simulink model "remote"  (Simulink 7.6)
settings: Solver=ode5  StartTime=0.0  StopTime=10.0  FixedStep=Ts  RelTol=1e-3
values from neighbouring files (symbols this model uses):
  g = 9.8065    [kostas_malakies.mat]    (also in kostas_malakies2.mat; load_PMModel.m = 9.81; main.m; main_last.m)
  mass = 0.66    [kostas_malakies.mat]    (also in kostas_malakies2.mat; load_PMModel.m = 0.687; main_last.m)
  N = 5    [matlab.mat]
  Ts = 0.02    [kostas_malakies.mat]    (also in kostas_malakies2.mat; main.m; main_last.m; matlab.mat = 0.08)
  Ts_slow = 0.02    [kostas_malakies.mat]    (also in kostas_malakies2.mat; main.m; main_last.m)
  yaw0 = 0    [kostas_malakies.mat]    (also in kostas_malakies2.mat; main.m; main_last.m; matlab.mat = -0.0873)
undefined symbols (not defined in the file or in its folder): AA_delay_x, AA_delay_y, AA_delay_yaw, AA_delay_z, BB_delay_x, BB_delay_y, BB_delay_yaw, BB_delay_z, betas_x, betas_y, betas_yaw, betas_z, delay_steps_x, delay_steps_y, delay_steps_yaw, delay_steps_z, i_min_cs_pre_rough_x, i_min_cs_pre_rough_y, i_min_cs_pre_rough_yaw, i_min_cs_pre_rough_z, kalmf_bias_x, kalmf_bias_y, kalmf_bias_z, L_x, L_y, L_yaw, L_z, LL_PP_x, LL_PP_y, LL_PP_yaw, LL_PP_z, LL_ref_PP_x, LL_ref_PP_y, LL_ref_PP_yaw, LL_ref_PP_z, MM_x, MM_y, MM_yaw, MM_z, PP_x, PP_y, PP_yaw, PP_z, TT_PP_x, TT_PP_y, TT_PP_yaw, TT_PP_z, V_max_x, V_max_y, V_max_yaw, V_max_z
libraries: simulink x18, Hqaud_model_LIB_SI x5, Hquad_control_LIB_SI x1
(part 1 of 2)
settings Model: Creator=burrimi  LastModifiedBy=burrimi
settings DataIOCC: SaveOutput=off  SaveTime=off
settings OptimizationCC: ZeroExternalMemoryAtStartup=off  OptimizeModelRefInitCode=on  LifeSpan=1
settings HardwareCC: ProdIntDivRoundTo=Zero  ProdEndianess=LittleEndian  ProdHWDeviceType=Intel Pentium  TargetIntDivRoundTo=Zero  TargetEndianess=LittleEndian  TargetHWDeviceType=MATLAB Host
settings RTWCC: SystemTargetFile=ert.tlc  TemplateMakefile=ert_default_tmf  Description=Real-Time Workshop Embedded Coder  GenerateReport=on  ProcessScript=ert_make_rtw_hook  IncludeHyperlinkInReport=on  LaunchReport=on  TargetLang=C++ (Encapsulated)
settings ERTTargetCC: MultiwordLength=2048  GenerateSampleERTMain=on  MultiInstanceERTCode=on  SupportContinuousTime=on  RootIOFormat=Structure reference  ERTCustomFileTemplate=example_file_process.tlc  ConvertIfToSwitch=off
settings ERTCPPComponent: GenerateDestructor=on  GenerateExternalIOAccessMethods=None  ParameterMemberVisibility=private  InternalMemberVisibility=private  GenerateParameterAccessMethods=None  GenerateInternalMemberAccessMethods=None  UseOperatorNewForModelRefRegistration=off

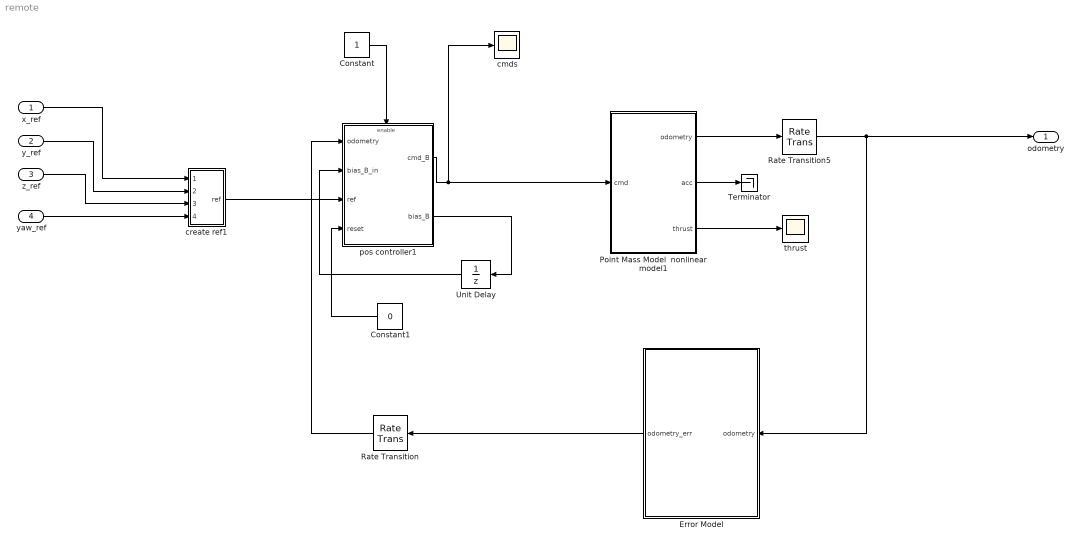
== system remote ==
  x_ref : Inport  PortDimensions=1  SampleTime=Ts
  y_ref : Inport  Port=2  PortDimensions=1  SampleTime=Ts
  z_ref : Inport  Port=3  PortDimensions=1  SampleTime=Ts
  yaw_ref : Inport  Port=4  PortDimensions=1  SampleTime=Ts
  Constant : Constant
  Constant1 : Constant  Value=0
  Error Model : Subsystem
  Point Mass Model  nonlinear model1 : Subsystem  AncestorBlock="Hqaud_model_LIB_SI/Point Mass Model  nonlinear model"
  Rate Transition : RateTransition  OutPortSampleTime=Ts
  Rate Transition5 : RateTransition  OutPortSampleTime=Ts_slow
  Terminator : Terminator
  Unit Delay : UnitDelay  SampleTime=-1
  cmds : Scope
      settings: TimeRange=39.996  YMin=-3  YMax=1
  create ref1 : Subsystem
  pos controller1 : Subsystem  AncestorBlock=Hquad_control_LIB_SI/pos controller
  thrust : Scope
      settings: TimeRange=40  YMin=113.9130434782609  YMax=138.2608695652174
  odometry : Outport  SampleTime=Ts
  wires:
  Point Mass Model  nonlinear model1/3("thrust   ") -> thrust/1
  pos controller1/1(cmd_B) -> cmds/1, Point Mass Model  nonlinear model1/1(cmd)
  Constant/1 -> pos controller1/Enable
  Point Mass Model  nonlinear model1/2(acc) -> Terminator/1
  Constant1/1 -> pos controller1/4(reset)
  Point Mass Model  nonlinear model1/1(odometry) -> Rate Transition5/1
  Rate Transition/1 -> pos controller1/1(odometry)
  Rate Transition5/1 -> odometry/1, Error Model/1(odometry)
  x_ref/1 -> create ref1/1(x_ref)
  y_ref/1 -> create ref1/2(y_ref)
  z_ref/1 -> create ref1/3(z_ref)
  yaw_ref/1 -> create ref1/4(yaw_ref)
  create ref1/1(ref) -> pos controller1/3(ref)
  pos controller1/2(bias_B) -> Unit Delay/1
  Unit Delay/1 -> pos controller1/2(bias_B_in)
  Error Model/1(odometry_err) -> Rate Transition/1

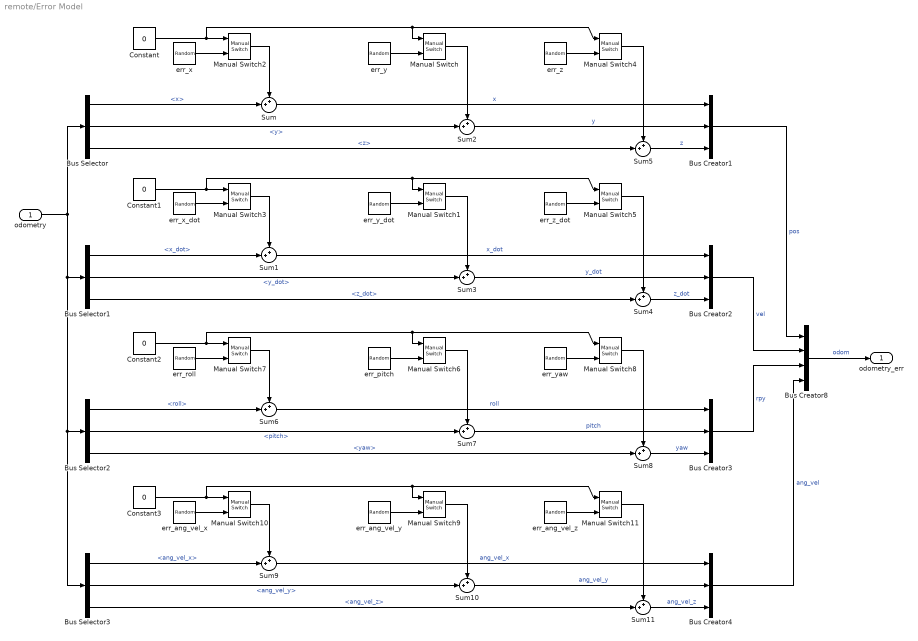
== system remote/Error Model ==
  odometry : Inport
  Bus Creator{1..4} (4 alike) : BusCreator  Inputs=3
  Bus Creator8 : BusCreator
  Bus Selector : BusSelector  OutputSignals=pos.x,pos.y,pos.z
  Bus Selector1 : BusSelector  OutputSignals=vel.x_dot,vel.y_dot,vel.z_dot
  Bus Selector2 : BusSelector  OutputSignals=rpy.roll,rpy.pitch,rpy.yaw
  Bus Selector3 : BusSelector  OutputSignals=ang_vel.ang_vel_x,ang_vel.ang_vel_y,ang_vel.ang_vel_z
  Constant{,1..3} (4 alike) : Constant  Value=0
  Manual Switch{,1..11} (12 alike) : simulink/Signal Routing/Manual Switch  SystemSampleTime=-1  sw=1  action=0  varsize=off
  Sum{,1..11} (12 alike) : Sum  Inputs=++|  SampleTime=Ts_slow
  err_ang_vel_x : RandomNumber  Variance=0.0001  SampleTime=Ts_slow
  err_ang_vel_y : RandomNumber  Variance=0.0001  SampleTime=Ts_slow
  err_ang_vel_z : RandomNumber  Variance=0.0001  SampleTime=Ts_slow
  err_pitch : RandomNumber  Variance=0.0001  SampleTime=Ts_slow
  err_roll : RandomNumber  Variance=0.0001  SampleTime=Ts_slow
  err_x : RandomNumber  Variance=0.000707  SampleTime=Ts_slow
  err_x_dot : RandomNumber  Variance=0.0001  SampleTime=Ts_slow
  err_y : RandomNumber  Variance=0.000707  SampleTime=Ts_slow
  err_y_dot : RandomNumber  Variance=0.0001  SampleTime=Ts_slow
  err_yaw : RandomNumber  Variance=0.0001  SampleTime=Ts_slow
  err_z : RandomNumber  Variance=0.000707  SampleTime=Ts_slow
  err_z_dot : RandomNumber  Variance=0.0001  SampleTime=Ts_slow
  odometry_err : Outport
  wires:
  err_z/1 -> Manual Switch4/2
  Manual Switch4/1 -> Sum5/1
  err_y/1 -> Manual Switch/2
  Manual Switch/1 -> Sum2/1
  err_x/1 -> Manual Switch2/2
  Manual Switch2/1 -> Sum/1
  Sum/1 -> Bus Creator1/1  "x"
  Bus Creator1/1 -> Bus Creator8/1  "pos"
  Sum2/1 -> Bus Creator1/2  "y"
  Sum5/1 -> Bus Creator1/3  "z"
  odometry/1 -> Bus Selector/1, Bus Selector2/1, Bus Selector3/1, Bus Selector1/1
  Bus Selector/1 -> Sum/2  "<x>"
  Bus Selector/2 -> Sum2/2  "<y>"
  Bus Selector/3 -> Sum5/2  "<z>"
  Constant/1 -> Manual Switch2/1, Manual Switch/1, Manual Switch4/1
  err_z_dot/1 -> Manual Switch5/2
  Manual Switch5/1 -> Sum4/1
  err_y_dot/1 -> Manual Switch1/2
  Manual Switch1/1 -> Sum3/1
  err_x_dot/1 -> Manual Switch3/2
  Manual Switch3/1 -> Sum1/1
  Sum1/1 -> Bus Creator2/1  "x_dot"
  Sum3/1 -> Bus Creator2/2  "y_dot"
  Sum4/1 -> Bus Creator2/3  "z_dot"
  Bus Selector1/1 -> Sum1/2  "<x_dot>"
  Bus Selector1/2 -> Sum3/2  "<y_dot>"
  Bus Selector1/3 -> Sum4/2  "<z_dot>"
  Constant1/1 -> Manual Switch3/1, Manual Switch1/1, Manual Switch5/1
  Bus Creator2/1 -> Bus Creator8/2  "vel"
  err_yaw/1 -> Manual Switch8/2
  Manual Switch8/1 -> Sum8/1
  err_pitch/1 -> Manual Switch6/2
  Manual Switch6/1 -> Sum7/1
  err_roll/1 -> Manual Switch7/2
  Manual Switch7/1 -> Sum6/1
  Sum6/1 -> Bus Creator3/1  "roll"
  Sum7/1 -> Bus Creator3/2  "pitch"
  Sum8/1 -> Bus Creator3/3  "yaw"
  Bus Selector2/1 -> Sum6/2  "<roll>"
  Bus Selector2/2 -> Sum7/2  "<pitch>"
  Bus Selector2/3 -> Sum8/2  "<yaw>"
  Constant2/1 -> Manual Switch7/1, Manual Switch6/1, Manual Switch8/1
  Bus Creator3/1 -> Bus Creator8/3  "rpy"
  err_ang_vel_z/1 -> Manual Switch11/2
  Manual Switch11/1 -> Sum11/1
  err_ang_vel_y/1 -> Manual Switch9/2
  Manual Switch9/1 -> Sum10/1
  err_ang_vel_x/1 -> Manual Switch10/2
  Manual Switch10/1 -> Sum9/1
  Sum9/1 -> Bus Creator4/1  "ang_vel_x"
  Sum10/1 -> Bus Creator4/2  "ang_vel_y"
  Sum11/1 -> Bus Creator4/3  "ang_vel_z"
  Bus Selector3/1 -> Sum9/2  "<ang_vel_x>"
  Bus Selector3/2 -> Sum10/2  "<ang_vel_y>"
  Bus Selector3/3 -> Sum11/2  "<ang_vel_z>"
  Constant3/1 -> Manual Switch10/1, Manual Switch9/1, Manual Switch11/1
  Bus Creator4/1 -> Bus Creator8/4  "ang_vel"
  Bus Creator8/1 -> odometry_err/1  "odom"

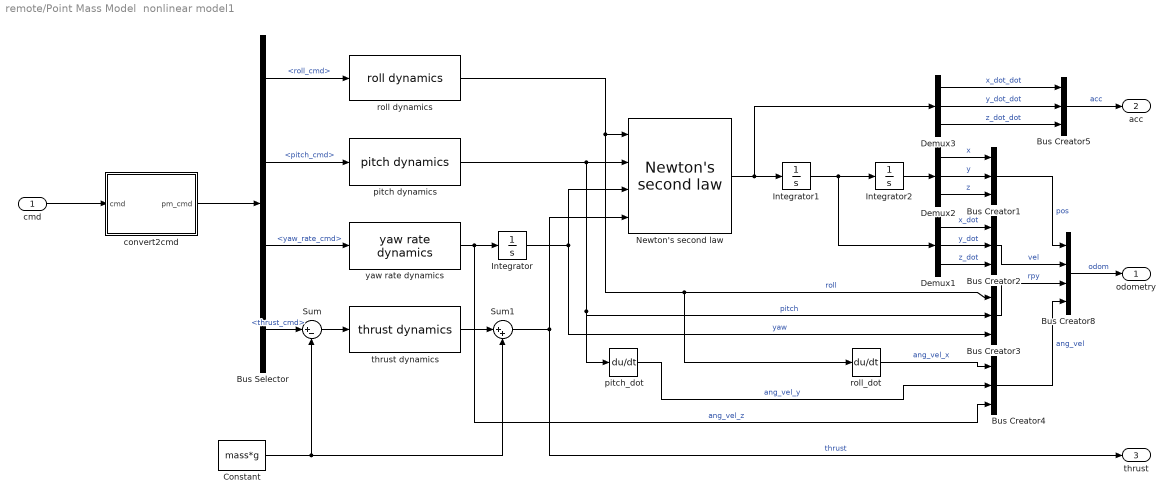
== system remote/Point Mass Model  nonlinear model1 ==
  cmd : Inport
  Bus Creator{1..5} (5 alike) : BusCreator  Inputs=3
  Bus Creator8 : BusCreator
  Bus Selector : BusSelector  OutputSignals=roll_cmd,pitch_cmd,yaw_rate_cmd,thrust_cmd
  Constant : Constant  Value=mass*g
  Demux1 : Demux  Outputs=3
  Demux2 : Demux  Outputs=3
  Demux3 : Demux  Outputs=3
  Integrator : Integrator  InitialCondition=yaw0
  Integrator1 : Integrator
  Integrator2 : Integrator
  "Newton's second law  " : Hqaud_model_LIB_SI/Newton's second law    SystemSampleTime=-1
  Sum : Sum  Inputs=|+-
  Sum1 : Sum  Inputs=|++
  convert2cmd : Subsystem
  "pitch dynamics  " : Hqaud_model_LIB_SI/pitch dynamics    SystemSampleTime=-1
  pitch_dot : Derivative
  roll dynamics : Hqaud_model_LIB_SI/roll dynamics  SystemSampleTime=-1
  roll_dot : Derivative
  "thrust dynamics  " : Hqaud_model_LIB_SI/thrust dynamics    SystemSampleTime=-1
  "yaw rate dynamics  " : Hqaud_model_LIB_SI/yaw rate dynamics    SystemSampleTime=-1
  odometry : Outport
  acc : Outport  Port=2
  "thrust   " : Outport  Port=3  PortDimensions=1
  wires:
  convert2cmd/1(pm_cmd) -> Bus Selector/1
  Bus Selector/1 -> roll dynamics/1  "<roll_cmd>"
  "yaw rate dynamics  "/1 -> Integrator/1, Bus Creator4/3  "ang_vel_z"
  Integrator/1 -> "Newton's second law  "/3, Bus Creator3/3  "yaw"
  "thrust dynamics  "/1 -> Sum1/1
  "pitch dynamics  "/1 -> "Newton's second law  "/2, Bus Creator3/2, pitch_dot/1  "pitch"
  roll dynamics/1 -> "Newton's second law  "/1, Bus Creator3/1, roll_dot/1  "roll"
  "Newton's second law  "/1 -> Integrator1/1, Demux3/1
  Integrator1/1 -> Integrator2/1, Demux1/1
  Integrator2/1 -> Demux2/1
  Demux2/2 -> Bus Creator1/2  "y"
  Constant/1 -> Sum/2, Sum1/2
  Sum/1 -> "thrust dynamics  "/1
  Bus Selector/4 -> Sum/1  "<thrust_cmd>"
  cmd/1 -> convert2cmd/1(cmd)
  Bus Selector/2 -> "pitch dynamics  "/1  "<pitch_cmd>"
  Bus Selector/3 -> "yaw rate dynamics  "/1  "<yaw_rate_cmd>"
  Bus Creator4/1 -> Bus Creator8/4  "ang_vel"
  Bus Creator3/1 -> Bus Creator8/3  "rpy"
  Bus Creator2/1 -> Bus Creator8/2  "vel"
  Bus Creator1/1 -> Bus Creator8/1  "pos"
  Bus Creator8/1 -> odometry/1  "odom"
  Demux2/3 -> Bus Creator1/3  "z"
  Demux2/1 -> Bus Creator1/1  "x"
  Demux1/1 -> Bus Creator2/1  "x_dot"
  Demux1/2 -> Bus Creator2/2  "y_dot"
  Demux1/3 -> Bus Creator2/3  "z_dot"
  Bus Creator5/1 -> acc/1  "acc"
  Demux3/1 -> Bus Creator5/1  "x_dot_dot"
  Demux3/2 -> Bus Creator5/2  "y_dot_dot"
  Demux3/3 -> Bus Creator5/3  "z_dot_dot"
  Sum1/1 -> "Newton's second law  "/4, "thrust   "/1  "thrust"
  roll_dot/1 -> Bus Creator4/1  "ang_vel_x"
  pitch_dot/1 -> Bus Creator4/2  "ang_vel_y"

== system remote/create ref1 ==
  x_ref : Inport
  y_ref : Inport  Port=2
  z_ref : Inport  Port=3
  yaw_ref : Inport  Port=4
  Bus Creator8 : BusCreator
  generate_X_ref : Stateflow chart  TreatAsAtomicUnit=on
  generate_X_ref1 : Stateflow chart  TreatAsAtomicUnit=on
  generate_X_ref2 : Stateflow chart  TreatAsAtomicUnit=on
  generate_X_ref3 : Stateflow chart  TreatAsAtomicUnit=on
  v_ref{1..4} (4 alike) : Constant  Value=0  OutDataTypeStr=double  SampleTime=-1
  ref : Outport
  wires:
  Bus Creator8/1 -> ref/1  "ref"
  generate_X_ref/1(X_ref) -> Bus Creator8/1  "X_ref_x"
  v_ref4/1 -> generate_X_ref/2(x_dot_ref)
  generate_X_ref1/1(X_ref) -> Bus Creator8/2  "X_ref_y"
  v_ref3/1 -> generate_X_ref1/2(x_dot_ref)  "x_dot_ref"
  generate_X_ref2/1(X_ref) -> Bus Creator8/3  "X_ref_z"
  v_ref2/1 -> generate_X_ref3/2(x_dot_ref)
  v_ref1/1 -> generate_X_ref2/2(x_dot_ref)
  generate_X_ref3/1(X_ref) -> Bus Creator8/4  "X_ref_yaw"
  x_ref/1 -> generate_X_ref/1(x_ref)
  y_ref/1 -> generate_X_ref1/1(x_ref)
  z_ref/1 -> generate_X_ref2/1(x_ref)
  yaw_ref/1 -> generate_X_ref3/1(x_ref)

== system remote/pos controller1 ==
  odometry : Inport
  bias_B_in : Inport  Port=2
  ref : Inport  Port=3
  reset : Inport  Port=4
  Enable : EnablePort  StatesWhenEnabling=reset
  MAIN CONTROL LOOP : Subsystem  Priority=2  AncestorBlock=Hquad_control_LIB_SI/MAIN CONTROL LOOP  TreatAsAtomicUnit=on
  decoupling and rotation : Subsystem  Priority=3  AncestorBlock=Hquad_control_LIB_SI/MAIN CONTROL LOOP  TreatAsAtomicUnit=on
  get ref from vector : Subsystem
  view & log signals : Subsystem
  yaw_correction : Subsystem  Priority=1  AncestorBlock=Hquad_control_LIB_SI/yaw_correction
  cmd_B : Outport
  bias_B : Outport  Port=2
  wires:
  MAIN CONTROL LOOP/1(cmd_W) -> view & log signals/3(cmd), decoupling and rotation/2(cmd_W)
  odometry/1 -> yaw_correction/1(odometry), view & log signals/1(odometry)
  reset/1 -> MAIN CONTROL LOOP/4(reset)
  ref/1 -> get ref from vector/1(X_ref), MAIN CONTROL LOOP/3(ref)
  get ref from vector/1(ref) -> view & log signals/2(ref)
  yaw_correction/1(odometry_rot) -> MAIN CONTROL LOOP/1(odometry), decoupling and rotation/1(odometry)
  MAIN CONTROL LOOP/2(bias_W_out) -> decoupling and rotation/3(bias_W)
  decoupling and rotation/1(cmd_B) -> cmd_B/1
  decoupling and rotation/2(bias_B) -> bias_B/1
  yaw_correction/2(bias_W) -> MAIN CONTROL LOOP/2(bias_W)
  bias_B_in/1 -> yaw_correction/2(bias_B)

== system remote/Point Mass Model  nonlinear model1/convert2cmd ==
  cmd : Inport
  Bus Creator8 : BusCreator
  Bus Selector : BusSelector  OutputSignals=pitch_cmd,roll_cmd,thrust_cmd,yaw_rate_cmd
  Sum : Sum  Inputs=++|
  Sum1 : Sum  Inputs=++|
  Sum2 : Sum  Inputs=++|
  offset pitch : Constant  Value=0/180*pi
  offset roll : Constant  Value=0/180*pi
  offset thrust : Constant  Value=0
  pm_cmd : Outport
  wires:
  Bus Selector/4 -> Bus Creator8/4  "<yaw_rate_cmd>"
  cmd/1 -> Bus Selector/1
  Bus Creator8/1 -> pm_cmd/1
  offset pitch/1 -> Sum/1
  Bus Selector/1 -> Sum/2  "<pitch_cmd>"
  Sum/1 -> Bus Creator8/1  "pitch_cmd"
  Bus Selector/3 -> Sum1/2  "<thrust_cmd>"
  Sum1/1 -> Bus Creator8/3  "thrust_cmd"
  offset thrust/1 -> Sum1/1
  Sum2/1 -> Bus Creator8/2  "roll_cmd"
  Bus Selector/2 -> Sum2/2  "<roll_cmd>"
  offset roll/1 -> Sum2/1

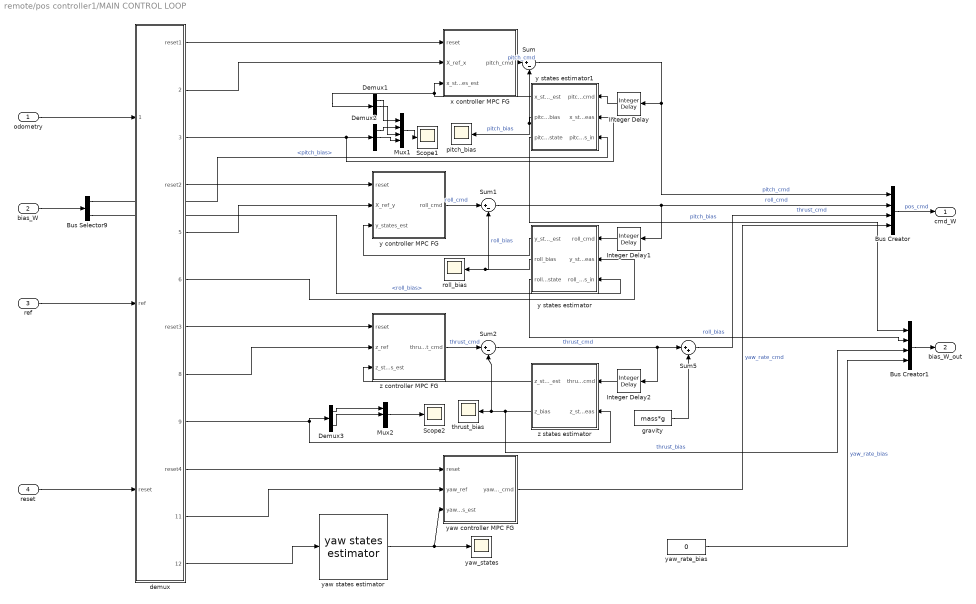
== system remote/pos controller1/MAIN CONTROL LOOP ==
  odometry : Inport
  bias_W : Inport  Port=2
  ref : Inport  Port=3
  reset : Inport  Port=4
  Bus Creator : BusCreator
  Bus Creator1 : BusCreator
  Bus Selector9 : BusSelector  OutputSignals=pitch_bias,roll_bias
  Demux1 : Demux  Outputs=3
  Demux2 : Demux  Outputs=3
  Demux3 : Demux  Outputs=2
  Integer Delay : simulink/Discrete/Integer Delay  NumDelays=delay_steps_x  vinit=0.0  samptime=-1
  Integer Delay1 : simulink/Discrete/Integer Delay  NumDelays=delay_steps_y  vinit=0.0  samptime=-1
  Integer Delay2 : simulink/Discrete/Integer Delay  NumDelays=delay_steps_z  vinit=0.0  samptime=-1
  Mux1 : Mux
  Mux2 : Mux  Inputs=5
  Scope1 : Scope
      settings: YMin=-0.2  YMax=1.3  SaveName=ScopeData6
  Scope2 : Scope
      settings: YMin=-0.4  YMax=1.4  SaveName=ScopeData15
  Sum : Sum  Inputs=|+-
  Sum1 : Sum  Inputs=|+-
  Sum2 : Sum  Inputs=|+-
  Sum5 : Sum  Inputs=|++
  demux : Subsystem
  gravity : Constant  Value=mass*g
  pitch_bias : Scope
      settings: YMin=-0.2  YMax=1.3  SaveName=ScopeData7
  roll_bias : Scope
      settings: YMin=-0.01  YMax=0.008  SaveName=ScopeData12
  thrust_bias : Scope
      settings: YMin=-0.0014  YMax=0.0001  SaveName=ScopeData13
  "x controller MPC FG  " : Subsystem
  y controller MPC FG : Subsystem
  y states estimator : Subsystem  AncestorBlock=Hquad_control_LIB_SI/x states estimator
  y states estimator1 : Subsystem  AncestorBlock=Hquad_control_LIB_SI/x states estimator
  yaw controller MPC FG : Subsystem
  yaw states estimator : Hquad_control_LIB_SI/yaw states estimator  SystemSampleTime=-1
  yaw_rate_bias : Constant  Value=0
  yaw_states : Scope
      settings: YMin=-0.4  YMax=1.4  SaveName=ScopeData16
  z controller MPC FG : Subsystem
  z states estimator : Subsystem  AncestorBlock=Hquad_control_LIB_SI/x states estimator
  cmd_W : Outport
  bias_W_out : Outport  Port=2
  wires:
  demux/11(X_ref_yaw) -> yaw controller MPC FG/2("yaw_ref  ")
  demux/9(z_states_meas) -> Demux3/1, z states estimator/2(z_states_meas)
  demux/6(y_states_meas) -> y states estimator/2(y_states_meas)
  demux/3(x_states_meas) -> Demux2/1, y states estimator1/2(x_states_meas)
  Bus Creator/1 -> cmd_W/1  "pos_cmd"
  demux/10(reset4) -> yaw controller MPC FG/1(reset)
  demux/7(reset3) -> z controller MPC FG/1(reset)
  demux/5(X_ref_y) -> y controller MPC FG/2("X_ref_y  ")
  demux/4(reset2) -> y controller MPC FG/1(reset)
  demux/1(reset1) -> "x controller MPC FG  "/1(reset)
  reset/1 -> demux/3(reset)
  ref/1 -> demux/2(ref)
  odometry/1 -> demux/1(odometry)
  demux/12(yaw_states_meas) -> yaw states estimator/1
  Integer Delay2/1 -> z states estimator/1(thrust_cmd)
  Integer Delay1/1 -> y states estimator/1(roll_cmd)
  demux/2(X_ref_x) -> "x controller MPC FG  "/2("X_ref_x  ")
  demux/8(X_ref_z) -> z controller MPC FG/2("z_ref  ")
  z states estimator/1(z_states_est) -> z controller MPC FG/3("z_states_est  ")
  Mux2/1 -> Scope2/1
  Demux3/1 -> Mux2/1
  Demux3/2 -> Mux2/3
  yaw states estimator/1 -> yaw_states/1, yaw controller MPC FG/3("yaw_states_est  ")
  Integer Delay/1 -> y states estimator1/1(pitch_cmd)
  y states estimator1/1(x_states_est) -> "x controller MPC FG  "/3("x_states_est  "), Demux1/1
  y states estimator/1(y_states_est) -> y controller MPC FG/3("y_states_est  ")
  yaw controller MPC FG/1("yaw_rate_cmd   ") -> Bus Creator/4  "yaw_rate_cmd"
  Demux1/1 -> Mux1/1
  Demux2/1 -> Mux1/2
  Demux1/2 -> Mux1/3
  Demux2/2 -> Mux1/4
  Mux1/1 -> Scope1/1
  "x controller MPC FG  "/1("pitch_cmd   ") -> Sum/1  "pitch_cmd"
  Sum/1 -> Integer Delay/1, Bus Creator/1  "pitch_cmd"
  y states estimator1/2(pitch_bias) -> pitch_bias/1, Sum/2  "pitch_bias"
  y controller MPC FG/1("roll_cmd   ") -> Sum1/1  "roll_cmd"
  Sum1/1 -> Integer Delay1/1, Bus Creator/2  "roll_cmd"
  y states estimator/2(roll_bias) -> roll_bias/1, Sum1/2  "roll_bias"
  z states estimator/2(z_bias) -> thrust_bias/1, Sum2/2, Bus Creator1/3  "thrust_bias"
  z controller MPC FG/1("thrust_cmd   ") -> Sum2/1  "thrust_cmd"
  Sum2/1 -> Integer Delay2/1, Sum5/1  "thrust_cmd"
  Bus Creator1/1 -> bias_W_out/1
  yaw_rate_bias/1 -> Bus Creator1/4  "yaw_rate_bias"
  gravity/1 -> Sum5/2
  Sum5/1 -> Bus Creator/3  "thrust_cmd"
  bias_W/1 -> Bus Selector9/1
  Bus Selector9/2 -> y states estimator/3(roll_bias_in)  "<roll_bias>"
  Bus Selector9/1 -> y states estimator1/3(pitch_bias_in)  "<pitch_bias>"
  y states estimator/3(roll_bias_state) -> Bus Creator1/2  "roll_bias"
  y states estimator1/3(pitch_bias_state) -> Bus Creator1/1  "pitch_bias"

== system remote/pos controller1/decoupling and rotation ==
  note: 
  odometry : Inport
  cmd_W : Inport  Port=2
  bias_W : Inport  Port=3
  Bus Selector1 : BusSelector  OutputSignals=rpy.yaw
  Bus Selector2 : BusSelector  OutputSignals=rpy.roll,rpy.pitch
  "decoupling " : Subsystem
  rotate_to_quat_frame : Subsystem
  cmd_B : Outport
  bias_B : Outport  Port=2
  wires:
  Bus Selector2/2 -> "decoupling "/2("pitch_meas  ")  "<pitch>"
  Bus Selector2/1 -> "decoupling "/1("roll_meas  ")  "<roll>"
  cmd_W/1 -> "decoupling "/3(cmd)
  bias_W/1 -> rotate_to_quat_frame/3(bias)
  rotate_to_quat_frame/2(bias_rot) -> bias_B/1
  Bus Selector1/1 -> rotate_to_quat_frame/1(yaw_meas)  "<yaw>"
  odometry/1 -> Bus Selector2/1, Bus Selector1/1
  "decoupling "/1("cmd_comp  ") -> rotate_to_quat_frame/2(cmd_comp)  "thrust_cmd"
  rotate_to_quat_frame/1("cmd_rot  ") -> cmd_B/1  "roll_cmd"

== system remote/pos controller1/get ref from vector ==
  X_ref : Inport
  Bus Creator2 : BusCreator
  Bus Creator3 : BusCreator
  Bus Creator4 : BusCreator  Inputs=2
  Bus Selector : BusSelector  OutputSignals=X_ref_x,X_ref_y,X_ref_z,X_ref_yaw
  Demux{1..4} (4 alike) : Demux  Outputs=2
  Selector{,1..3} (4 alike) : Selector  IndexOptions=Index vector (dialog)  Indices=[1 2]  OutputSizes=1
  ref : Outport
  wires:
  X_ref/1 -> Bus Selector/1
  Bus Selector/1 -> Selector/1  "<X_ref_x>"
  Bus Selector/4 -> Selector3/1  "<X_ref_yaw>"
  Bus Selector/3 -> Selector2/1  "<X_ref_z>"
  Bus Selector/2 -> Selector1/1  "<X_ref_y>"
  Selector/1 -> Demux1/1
  Selector3/1 -> Demux4/1
  Selector2/1 -> Demux3/1
  Selector1/1 -> Demux2/1
  Bus Creator2/1 -> Bus Creator4/1  "pose_ref"
  Bus Creator3/1 -> Bus Creator4/2  "vel_ref"
  Bus Creator4/1 -> ref/1  "ref"
  Demux1/1 -> Bus Creator2/1  "x_ref"
  Demux2/1 -> Bus Creator2/2  "y_ref"
  Demux3/1 -> Bus Creator2/3  "z_ref"
  Demux4/1 -> Bus Creator2/4  "yaw_ref"
  Demux1/2 -> Bus Creator3/1  "x_dot_ref"
  Demux2/2 -> Bus Creator3/2  "y_dot_ref"
  Demux3/2 -> Bus Creator3/3  "z_dot_ref"
  Demux4/2 -> Bus Creator3/4  "yaw_dot_ref"

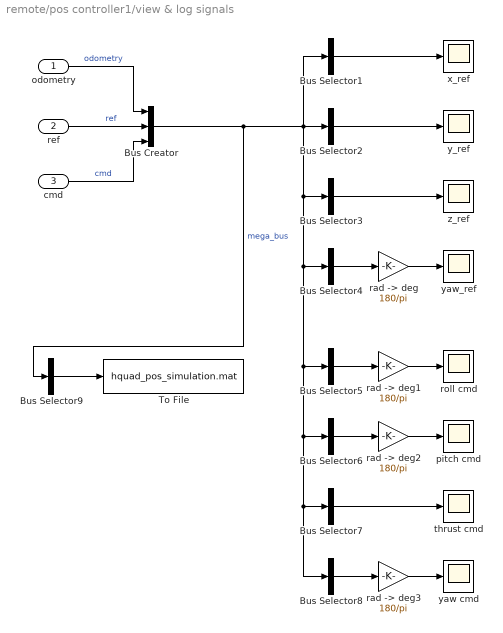
== system remote/pos controller1/view & log signals ==
  odometry : Inport
  ref : Inport  Port=2
  cmd : Inport  Port=3
  Bus Creator : BusCreator  Inputs=3
  Bus Selector1 : BusSelector  OutputSignals=odometry.pos.x,odometry.vel.x_dot,ref.pose_ref.x_ref,ref.vel_ref.x_dot_ref  OutputAsBus=on
  Bus Selector2 : BusSelector  OutputSignals=odometry.pos.y,odometry.vel.y_dot,ref.pose_ref.y_ref,ref.vel_ref.y_dot_ref  OutputAsBus=on
  Bus Selector3 : BusSelector  OutputSignals=odometry.pos.z,odometry.vel.z_dot,ref.pose_ref.z_ref,ref.vel_ref.z_dot_ref  OutputAsBus=on
  Bus Selector4 : BusSelector  OutputSignals=odometry.rpy.yaw,odometry.ang_vel.ang_vel_z,ref.pose_ref.yaw_ref,ref.vel_ref.yaw_dot_ref  OutputAsBus=on
  Bus Selector5 : BusSelector  OutputSignals=odometry.rpy.roll,odometry.ang_vel.ang_vel_x,cmd.roll_cmd  OutputAsBus=on
  Bus Selector6 : BusSelector  OutputSignals=odometry.rpy.pitch,odometry.ang_vel.ang_vel_y,cmd.pitch_cmd  OutputAsBus=on
  Bus Selector7 : BusSelector  OutputSignals=odometry.pos.z,ref.pose_ref.z_ref,cmd.thrust_cmd  OutputAsBus=on
  Bus Selector8 : BusSelector  OutputSignals=odometry.rpy.yaw,odometry.ang_vel.ang_vel_z,cmd.yaw_rate_cmd  OutputAsBus=on
  Bus Selector9 : BusSelector  OutputSignals=odometry.pos.x,odometry.vel.x_dot,odometry.rpy.pitch,ref.pose_ref.x_ref,cmd.pitch_cmd,odometry.pos.y,odometry.vel.y_dot,odometry.rpy.roll,ref.pose_ref.y_ref,cmd.roll_cmd,odometry.pos.z,odometry.vel.z_dot,ref.pose_ref.z_ref,cmd.thrust_cmd  OutputAsBus=on
  To File : ToFile  Filename=hquad_pos_simulation.mat  MatrixName=hquad_pos_simulation
  pitch cmd : Scope
      settings: YMin=-15  YMax=15  SaveName=ScopeData2
  rad -> deg{,1..3} (4 alike) : Gain  Gain=180/pi
  roll cmd : Scope
      settings: YMin=-100  YMax=100
  thrust cmd : Scope
      settings: YMin=-3  YMax=3  SaveName=ScopeData11
  x_ref : Scope
      settings: TimeRange=40  YMin=-1.5  YMax=1.5  SaveName=ScopeData3
  y_ref : Scope
      settings: TimeRange=40  YMin=-1.5  YMax=1.5
  yaw cmd : Scope
      settings: YMin=-60  YMax=-0  SaveName=ScopeData10
  yaw_ref : Scope
      settings: TimeRange=39.996  YMin=0  YMax=3250  SaveName=ScopeData8
  z_ref : Scope
      settings: YMin=-1.1  YMax=0.05  SaveName=ScopeData5
  wires:
  Bus Selector8/1 -> "rad -> deg3"/1
  Bus Selector6/1 -> "rad -> deg2"/1
  Bus Selector5/1 -> "rad -> deg1"/1
  Bus Selector7/1 -> thrust cmd/1
  Bus Selector4/1 -> "rad -> deg"/1
  Bus Selector3/1 -> z_ref/1
  Bus Selector2/1 -> y_ref/1
  Bus Selector1/1 -> x_ref/1
  Bus Creator/1 -> Bus Selector8/1, Bus Selector7/1, Bus Selector6/1, Bus Selector5/1, Bus Selector4/1, Bus Selector3/1, Bus Selector2/1, Bus Selector1/1, Bus Selector9/1  "mega_bus"
  cmd/1 -> Bus Creator/3  "cmd"
  ref/1 -> Bus Creator/2  "ref"
  odometry/1 -> Bus Creator/1  "odometry"
  "rad -> deg3"/1 -> yaw cmd/1
  "rad -> deg2"/1 -> pitch cmd/1
  "rad -> deg1"/1 -> roll cmd/1
  "rad -> deg"/1 -> yaw_ref/1
  Bus Selector9/1 -> To File/1

== system remote/pos controller1/yaw_correction ==
  odometry : Inport
  bias_B : Inport  Port=2
  Bus Creator1 : BusCreator  Inputs=3
  Bus Creator2 : BusCreator
  Bus Creator5 : BusCreator
  Bus Selector1 : BusSelector  OutputSignals=rpy.roll,rpy.pitch
  Bus Selector2 : BusSelector  OutputSignals=ang_vel
  Bus Selector3 : BusSelector  OutputSignals=rpy.yaw
  Bus Selector4 : BusSelector  OutputSignals=thrust_bias,yaw_rate_bias
  Bus Selector5 : BusSelector  OutputSignals=pitch_bias,roll_bias
  Bus Selector6 : BusSelector  OutputSignals=pos,vel
  Embedded MATLAB Function : Stateflow chart  TreatAsAtomicUnit=on
  odometry_rot : Outport
  bias_W : Outport  Port=2
  wires:
  Bus Selector6/2 -> Bus Creator5/2  "<vel>"
  Bus Selector6/1 -> Bus Creator5/1  "<pos>"
  Bus Creator5/1 -> odometry_rot/1  "odom"
  Bus Selector3/1 -> Embedded MATLAB Function/5(yaw), Bus Creator1/3  "<yaw>"
  odometry/1 -> Bus Selector3/1, Bus Selector1/1, Bus Selector6/1, Bus Selector2/1
  Bus Selector2/1 -> Bus Creator5/4  "<ang_vel>"
  Bus Creator1/1 -> Bus Creator5/3  "rpy"
  Embedded MATLAB Function/1(roll_rot) -> Bus Creator1/1  "roll"
  Embedded MATLAB Function/2(pitch_rot) -> Bus Creator1/2  "pitch"
  Bus Selector1/1 -> Embedded MATLAB Function/1(roll)  "<roll>"
  Bus Selector1/2 -> Embedded MATLAB Function/2(pitch)  "<pitch>"
  Bus Creator2/1 -> bias_W/1
  Bus Selector4/2 -> Bus Creator2/4  "<yaw_rate_bias>"
  Bus Selector4/1 -> Bus Creator2/3  "<thrust_bias>"
  Bus Selector5/1 -> Embedded MATLAB Function/3(pitch_bias)  "<pitch_bias>"
  Bus Selector5/2 -> Embedded MATLAB Function/4(roll_bias)  "<roll_bias>"
  bias_B/1 -> Bus Selector5/1, Bus Selector4/1
  Embedded MATLAB Function/3(pitch_bias_rot) -> Bus Creator2/1  "pitch_bias"
  Embedded MATLAB Function/4(roll_bias_rot) -> Bus Creator2/2  "roll_bias"

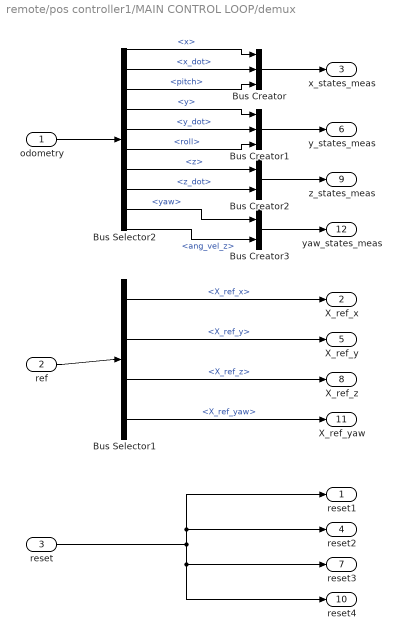
== system remote/pos controller1/MAIN CONTROL LOOP/demux ==
  odometry : Inport
  ref : Inport  Port=2
  reset : Inport  Port=3
  Bus Creator : BusCreator  Inputs=3
  Bus Creator1 : BusCreator  Inputs=3
  Bus Creator2 : BusCreator  Inputs=2
  Bus Creator3 : BusCreator  Inputs=2
  Bus Selector1 : BusSelector  OutputSignals=X_ref_x,X_ref_y,X_ref_z,X_ref_yaw
  Bus Selector2 : BusSelector  OutputSignals=pos.x,vel.x_dot,rpy.pitch,pos.y,vel.y_dot,rpy.roll,pos.z,vel.z_dot,rpy.yaw,ang_vel.ang_vel_z
  reset1 : Outport
  X_ref_x : Outport  Port=2
  x_states_meas : Outport  Port=3  PortDimensions=3
  reset2 : Outport  Port=4
  X_ref_y : Outport  Port=5
  y_states_meas : Outport  Port=6  PortDimensions=3
  reset3 : Outport  Port=7
  X_ref_z : Outport  Port=8
  z_states_meas : Outport  Port=9  PortDimensions=2
  reset4 : Outport  Port=10
  X_ref_yaw : Outport  Port=11
  yaw_states_meas : Outport  Port=12  PortDimensions=2
  wires:
  reset/1 -> reset1/1, reset2/1, reset4/1, reset3/1
  Bus Selector1/2 -> X_ref_y/1  "<X_ref_y>"
  Bus Selector1/1 -> X_ref_x/1  "<X_ref_x>"
  ref/1 -> Bus Selector1/1
  Bus Creator3/1 -> yaw_states_meas/1
  Bus Creator2/1 -> z_states_meas/1
  Bus Selector2/10 -> Bus Creator3/2  "<ang_vel_z>"
  Bus Selector2/9 -> Bus Creator3/1  "<yaw>"
  Bus Selector2/8 -> Bus Creator2/2  "<z_dot>"
  Bus Selector2/7 -> Bus Creator2/1  "<z>"
  Bus Creator1/1 -> y_states_meas/1
  Bus Selector2/5 -> Bus Creator1/2  "<y_dot>"
  Bus Selector2/4 -> Bus Creator1/1  "<y>"
  Bus Selector2/2 -> Bus Creator/2  "<x_dot>"
  Bus Selector2/1 -> Bus Creator/1  "<x>"
  Bus Creator/1 -> x_states_meas/1
  odometry/1 -> Bus Selector2/1
  Bus Selector2/3 -> Bus Creator/3  "<pitch>"
  Bus Selector2/6 -> Bus Creator1/3  "<roll>"
  Bus Selector1/3 -> X_ref_z/1  "<X_ref_z>"
  Bus Selector1/4 -> X_ref_yaw/1  "<X_ref_yaw>"

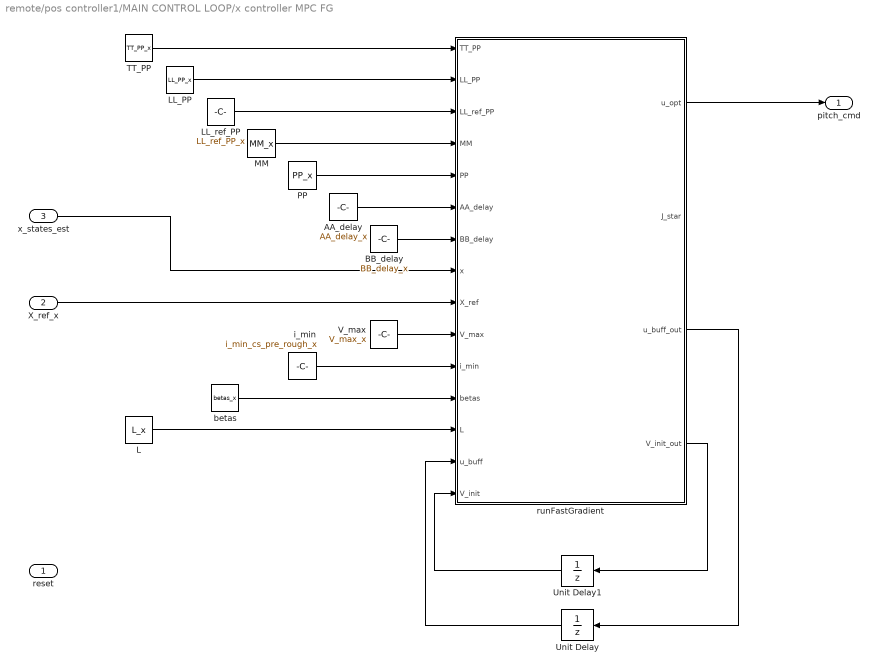
== system remote/pos controller1/MAIN CONTROL LOOP/x controller MPC FG   ==
  reset : Inport  PortDimensions=1
  "X_ref_x  " : Inport  Port=2
  "x_states_est  " : Inport  Port=3
  AA_delay : Constant  Value=AA_delay_x
  BB_delay : Constant  Value=BB_delay_x
  L : Constant  Value=L_x
  LL_PP : Constant  Value=LL_PP_x
  LL_ref_PP : Constant  Value=LL_ref_PP_x
  MM : Constant  Value=MM_x
  PP : Constant  Value=PP_x
  TT_PP : Constant  Value=TT_PP_x
  Unit Delay : UnitDelay  X0=zeros(delay_steps_x,1)  SampleTime=-1
  Unit Delay1 : UnitDelay  X0=zeros(N,1)  SampleTime=-1
  V_max : Constant  Value=V_max_x
  betas : Constant  Value=betas_x
  i_min : Constant  Value=i_min_cs_pre_rough_x
  runFastGradient : Stateflow chart  TreatAsAtomicUnit=on
  "pitch_cmd   " : Outport  PortDimensions=1
  wires:
  "x_states_est  "/1 -> runFastGradient/8(x)
  runFastGradient/1(u_opt) -> "pitch_cmd   "/1
  "X_ref_x  "/1 -> runFastGradient/9(X_ref)
  TT_PP/1 -> runFastGradient/1(TT_PP)
  LL_PP/1 -> runFastGradient/2(LL_PP)
  runFastGradient/4(V_init_out) -> Unit Delay1/1
  runFastGradient/3(u_buff_out) -> Unit Delay/1
  Unit Delay1/1 -> runFastGradient/15(V_init)
  Unit Delay/1 -> runFastGradient/14(u_buff)
  LL_ref_PP/1 -> runFastGradient/3(LL_ref_PP)
  MM/1 -> runFastGradient/4(MM)
  PP/1 -> runFastGradient/5(PP)
  AA_delay/1 -> runFastGradient/6(AA_delay)
  BB_delay/1 -> runFastGradient/7(BB_delay)
  V_max/1 -> runFastGradient/10(V_max)
  i_min/1 -> runFastGradient/11(i_min)
  betas/1 -> runFastGradient/12(betas)
  L/1 -> runFastGradient/13(L)

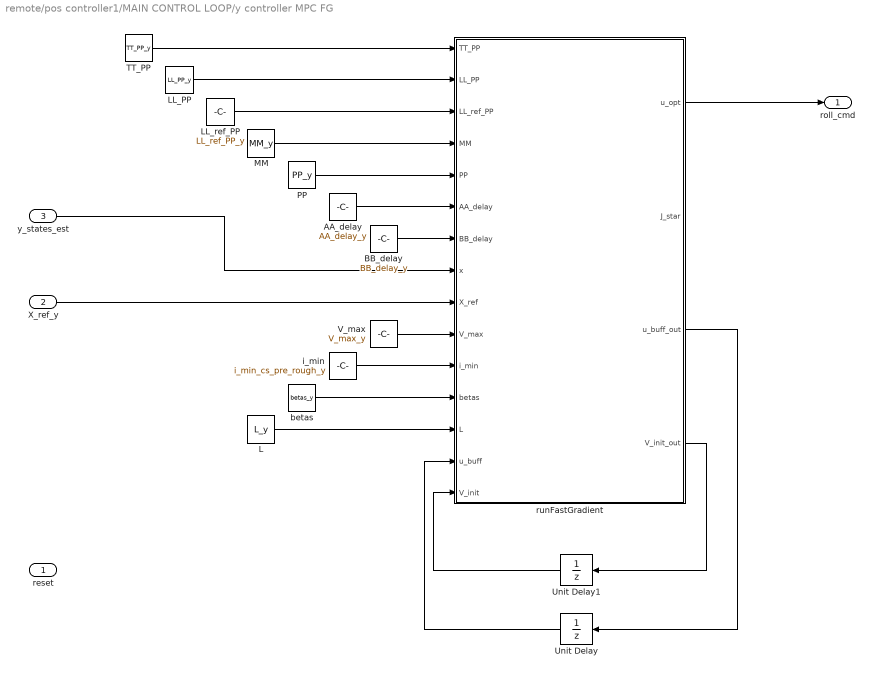
== system remote/pos controller1/MAIN CONTROL LOOP/y controller MPC FG ==
  reset : Inport  PortDimensions=1
  "X_ref_y  " : Inport  Port=2
  "y_states_est  " : Inport  Port=3
  AA_delay : Constant  Value=AA_delay_y
  BB_delay : Constant  Value=BB_delay_y
  L : Constant  Value=L_y
  LL_PP : Constant  Value=LL_PP_y
  LL_ref_PP : Constant  Value=LL_ref_PP_y
  MM : Constant  Value=MM_y
  PP : Constant  Value=PP_y
  TT_PP : Constant  Value=TT_PP_y
  Unit Delay : UnitDelay  X0=zeros(delay_steps_y,1)  SampleTime=-1
  Unit Delay1 : UnitDelay  X0=zeros(N,1)  SampleTime=-1
  V_max : Constant  Value=V_max_y
  betas : Constant  Value=betas_y
  i_min : Constant  Value=i_min_cs_pre_rough_y
  runFastGradient : Stateflow chart  TreatAsAtomicUnit=on
  "roll_cmd   " : Outport  PortDimensions=1
  wires:
  "y_states_est  "/1 -> runFastGradient/8(x)
  runFastGradient/1(u_opt) -> "roll_cmd   "/1
  "X_ref_y  "/1 -> runFastGradient/9(X_ref)
  TT_PP/1 -> runFastGradient/1(TT_PP)
  LL_PP/1 -> runFastGradient/2(LL_PP)
  runFastGradient/4(V_init_out) -> Unit Delay1/1
  runFastGradient/3(u_buff_out) -> Unit Delay/1
  Unit Delay1/1 -> runFastGradient/15(V_init)
  Unit Delay/1 -> runFastGradient/14(u_buff)
  LL_ref_PP/1 -> runFastGradient/3(LL_ref_PP)
  MM/1 -> runFastGradient/4(MM)
  PP/1 -> runFastGradient/5(PP)
  AA_delay/1 -> runFastGradient/6(AA_delay)
  BB_delay/1 -> runFastGradient/7(BB_delay)
  V_max/1 -> runFastGradient/10(V_max)
  i_min/1 -> runFastGradient/11(i_min)
  betas/1 -> runFastGradient/12(betas)
  L/1 -> runFastGradient/13(L)

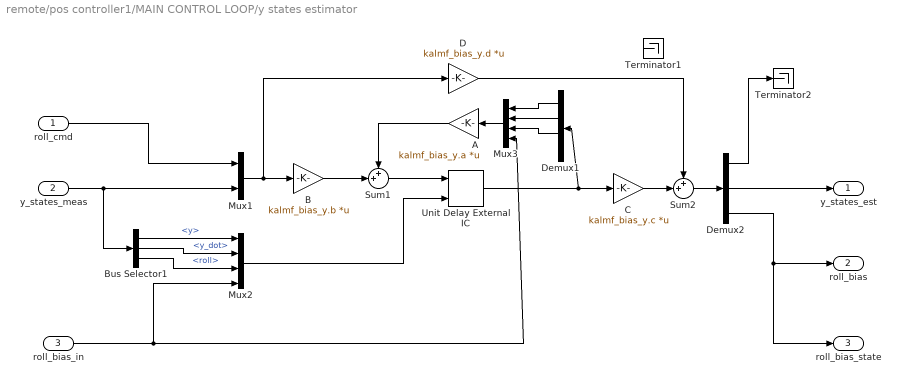
== system remote/pos controller1/MAIN CONTROL LOOP/y states estimator ==
  roll_cmd : Inport  PortDimensions=1
  y_states_meas : Inport  Port=2  PortDimensions=3
  roll_bias_in : Inport  Port=3  PortDimensions=1
  A : Gain  Gain=kalmf_bias_y.a  Multiplication=Matrix(K*u)  SampleTime=Ts
  B : Gain  Gain=kalmf_bias_y.b  Multiplication=Matrix(K*u)  SampleTime=Ts
  Bus Selector1 : BusSelector  OutputSignals=y,y_dot,roll
  C : Gain  Gain=kalmf_bias_y.c  Multiplication=Matrix(K*u)  SampleTime=Ts
  D : Gain  Gain=kalmf_bias_y.d  Multiplication=Matrix(K*u)  SampleTime=Ts
  Demux1 : Demux
  Demux2 : Demux  Outputs=3
  Mux1 : Mux  Inputs=2
  Mux2 : Mux
  Mux3 : Mux
  Sum1 : Sum  Inputs=++|
  Sum2 : Sum  Inputs=++|
  Terminator1 : Terminator
  Terminator2 : Terminator
  Unit Delay External IC : simulink/Additional Math & Discrete/Additional Discrete/Unit Delay External IC  SystemSampleTime=-1  tsamp=-1
  y_states_est : Outport  PortDimensions=3
  roll_bias : Outport  Port=2  PortDimensions=1
  roll_bias_state : Outport  Port=3  PortDimensions=1
  wires:
  Demux2/2 -> y_states_est/1
  Demux2/1 -> Terminator2/1
  y_states_meas/1 -> Bus Selector1/1, Mux1/2
  roll_cmd/1 -> Mux1/1
  Mux1/1 -> B/1, D/1
  Unit Delay External IC/1 -> C/1, Demux1/1
  Mux2/1 -> Unit Delay External IC/2
  A/1 -> Sum1/1
  C/1 -> Sum2/2
  D/1 -> Sum2/1
  B/1 -> Sum1/2
  Sum1/1 -> Unit Delay External IC/1
  Sum2/1 -> Demux2/1
  Mux3/1 -> A/1
  Demux1/1 -> Mux3/1
  Demux1/2 -> Mux3/2
  Demux1/3 -> Mux3/3
  roll_bias_in/1 -> Mux3/4, Mux2/4
  Bus Selector1/1 -> Mux2/1  "<y>"
  Bus Selector1/2 -> Mux2/2  "<y_dot>"
  Bus Selector1/3 -> Mux2/3  "<roll>"
  Demux2/3 -> roll_bias/1, roll_bias_state/1

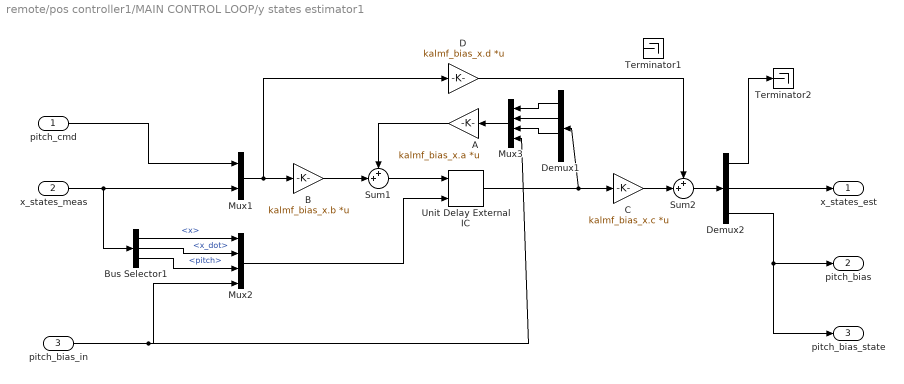
== system remote/pos controller1/MAIN CONTROL LOOP/y states estimator1 ==
  pitch_cmd : Inport  PortDimensions=1
  x_states_meas : Inport  Port=2  PortDimensions=3
  pitch_bias_in : Inport  Port=3  PortDimensions=1
  A : Gain  Gain=kalmf_bias_x.a  Multiplication=Matrix(K*u)  SampleTime=Ts
  B : Gain  Gain=kalmf_bias_x.b  Multiplication=Matrix(K*u)  SampleTime=Ts
  Bus Selector1 : BusSelector  OutputSignals=x,x_dot,pitch
  C : Gain  Gain=kalmf_bias_x.c  Multiplication=Matrix(K*u)  SampleTime=Ts
  D : Gain  Gain=kalmf_bias_x.d  Multiplication=Matrix(K*u)  SampleTime=Ts
  Demux1 : Demux
  Demux2 : Demux  Outputs=3
  Mux1 : Mux  Inputs=2
  Mux2 : Mux
  Mux3 : Mux
  Sum1 : Sum  Inputs=++|
  Sum2 : Sum  Inputs=++|
  Terminator1 : Terminator
  Terminator2 : Terminator
  Unit Delay External IC : simulink/Additional Math & Discrete/Additional Discrete/Unit Delay External IC  SystemSampleTime=-1  tsamp=-1
  x_states_est : Outport  PortDimensions=3
  pitch_bias : Outport  Port=2  PortDimensions=1
  pitch_bias_state : Outport  Port=3  PortDimensions=1
  wires:
  Demux2/2 -> x_states_est/1
  Demux2/1 -> Terminator2/1
  x_states_meas/1 -> Bus Selector1/1, Mux1/2
  pitch_cmd/1 -> Mux1/1
  Mux1/1 -> B/1, D/1
  Unit Delay External IC/1 -> C/1, Demux1/1
  Mux2/1 -> Unit Delay External IC/2
  A/1 -> Sum1/1
  C/1 -> Sum2/2
  D/1 -> Sum2/1
  B/1 -> Sum1/2
  Sum1/1 -> Unit Delay External IC/1
  Sum2/1 -> Demux2/1
  Demux2/3 -> pitch_bias/1, pitch_bias_state/1
  Mux3/1 -> A/1
  Demux1/1 -> Mux3/1
  Demux1/2 -> Mux3/2
  Demux1/3 -> Mux3/3
  pitch_bias_in/1 -> Mux2/4, Mux3/4
  Bus Selector1/1 -> Mux2/1  "<x>"
  Bus Selector1/2 -> Mux2/2  "<x_dot>"
  Bus Selector1/3 -> Mux2/3  "<pitch>"

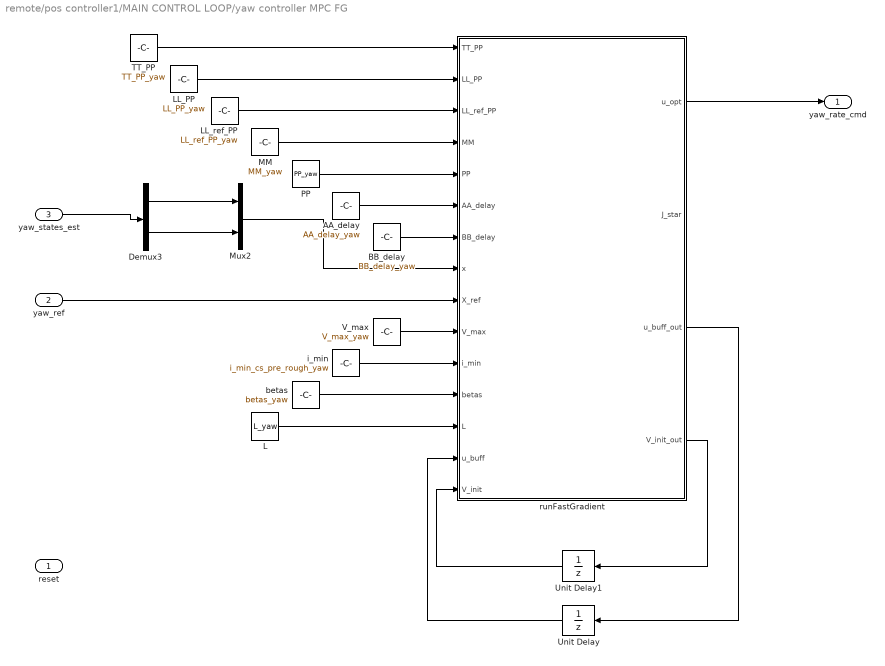
== system remote/pos controller1/MAIN CONTROL LOOP/yaw controller MPC FG ==
  reset : Inport  PortDimensions=1
  "yaw_ref  " : Inport  Port=2
  "yaw_states_est  " : Inport  Port=3
  AA_delay : Constant  Value=AA_delay_yaw
  BB_delay : Constant  Value=BB_delay_yaw
  Demux3 : Demux  Outputs=2
  L : Constant  Value=L_yaw
  LL_PP : Constant  Value=LL_PP_yaw
  LL_ref_PP : Constant  Value=LL_ref_PP_yaw
  MM : Constant  Value=MM_yaw
  Mux2 : Mux  Inputs=2
  PP : Constant  Value=PP_yaw
  TT_PP : Constant  Value=TT_PP_yaw
  Unit Delay : UnitDelay  X0=zeros(delay_steps_yaw,1)  SampleTime=-1
  Unit Delay1 : UnitDelay  X0=zeros(N,1)  SampleTime=-1
  V_max : Constant  Value=V_max_yaw
  betas : Constant  Value=betas_yaw
  i_min : Constant  Value=i_min_cs_pre_rough_yaw
  runFastGradient : Stateflow chart  TreatAsAtomicUnit=on
  "yaw_rate_cmd   " : Outport  PortDimensions=1
  wires:
  Demux3/1 -> Mux2/1
  "yaw_states_est  "/1 -> Demux3/1
  runFastGradient/1(u_opt) -> "yaw_rate_cmd   "/1
  "yaw_ref  "/1 -> runFastGradient/9(X_ref)
  Demux3/2 -> Mux2/2
  TT_PP/1 -> runFastGradient/1(TT_PP)
  LL_PP/1 -> runFastGradient/2(LL_PP)
  runFastGradient/4(V_init_out) -> Unit Delay1/1
  runFastGradient/3(u_buff_out) -> Unit Delay/1
  Unit Delay1/1 -> runFastGradient/15(V_init)
  Unit Delay/1 -> runFastGradient/14(u_buff)
  LL_ref_PP/1 -> runFastGradient/3(LL_ref_PP)
  MM/1 -> runFastGradient/4(MM)
  PP/1 -> runFastGradient/5(PP)
  AA_delay/1 -> runFastGradient/6(AA_delay)
  BB_delay/1 -> runFastGradient/7(BB_delay)
  Mux2/1 -> runFastGradient/8(x)
  V_max/1 -> runFastGradient/10(V_max)
  i_min/1 -> runFastGradient/11(i_min)
  betas/1 -> runFastGradient/12(betas)
  L/1 -> runFastGradient/13(L)

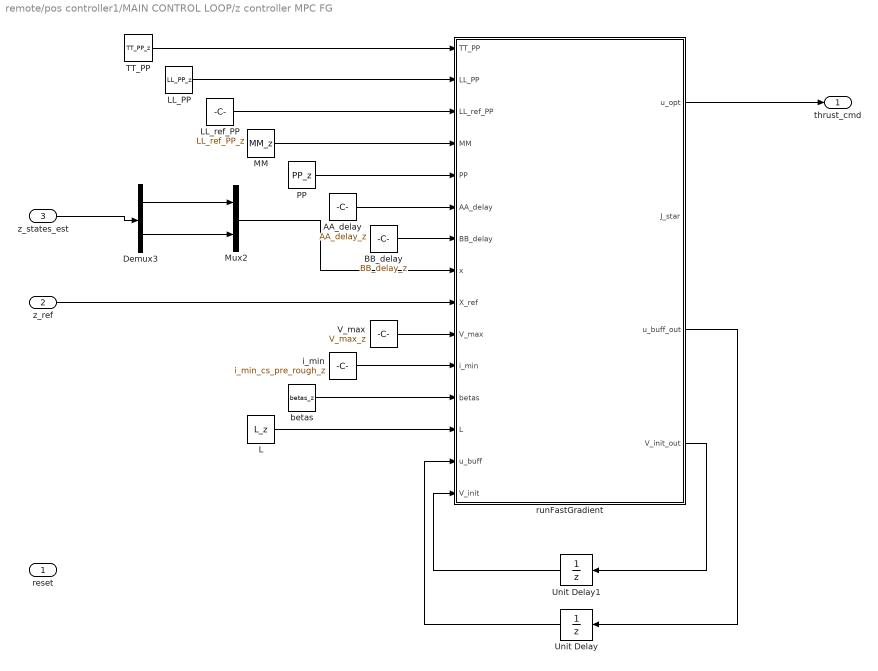
== system remote/pos controller1/MAIN CONTROL LOOP/z controller MPC FG ==
  reset : Inport  PortDimensions=1
  "z_ref  " : Inport  Port=2
  "z_states_est  " : Inport  Port=3
  AA_delay : Constant  Value=AA_delay_z
  BB_delay : Constant  Value=BB_delay_z
  Demux3 : Demux  Outputs=2
  L : Constant  Value=L_z
  LL_PP : Constant  Value=LL_PP_z
  LL_ref_PP : Constant  Value=LL_ref_PP_z
  MM : Constant  Value=MM_z
  Mux2 : Mux  Inputs=2
  PP : Constant  Value=PP_z
  TT_PP : Constant  Value=TT_PP_z
  Unit Delay : UnitDelay  X0=zeros(delay_steps_z,1)  SampleTime=-1
  Unit Delay1 : UnitDelay  X0=zeros(N,1)  SampleTime=-1
  V_max : Constant  Value=V_max_z
  betas : Constant  Value=betas_z
  i_min : Constant  Value=i_min_cs_pre_rough_z
  runFastGradient : Stateflow chart  TreatAsAtomicUnit=on
  "thrust_cmd   " : Outport  PortDimensions=1
  wires:
  Demux3/1 -> Mux2/1
  "z_states_est  "/1 -> Demux3/1
  runFastGradient/1(u_opt) -> "thrust_cmd   "/1
  "z_ref  "/1 -> runFastGradient/9(X_ref)
  Demux3/2 -> Mux2/2
  TT_PP/1 -> runFastGradient/1(TT_PP)
  LL_PP/1 -> runFastGradient/2(LL_PP)
  runFastGradient/4(V_init_out) -> Unit Delay1/1
  runFastGradient/3(u_buff_out) -> Unit Delay/1
  Unit Delay1/1 -> runFastGradient/15(V_init)
  Unit Delay/1 -> runFastGradient/14(u_buff)
  LL_ref_PP/1 -> runFastGradient/3(LL_ref_PP)
  MM/1 -> runFastGradient/4(MM)
  PP/1 -> runFastGradient/5(PP)
  AA_delay/1 -> runFastGradient/6(AA_delay)
  BB_delay/1 -> runFastGradient/7(BB_delay)
  Mux2/1 -> runFastGradient/8(x)
  V_max/1 -> runFastGradient/10(V_max)
  i_min/1 -> runFastGradient/11(i_min)
  betas/1 -> runFastGradient/12(betas)
  L/1 -> runFastGradient/13(L)

== system remote/pos controller1/MAIN CONTROL LOOP/z states estimator ==
  thrust_cmd : Inport  PortDimensions=1
  z_states_meas : Inport  Port=2  PortDimensions=2
  A : Gain  Gain=kalmf_bias_z.a  Multiplication=Matrix(K*u)  SampleTime=Ts
  B : Gain  Gain=kalmf_bias_z.b  Multiplication=Matrix(K*u)  SampleTime=Ts
  Bus Selector1 : BusSelector  OutputSignals=z,z_dot  OutputAsBus=on
  C : Gain  Gain=kalmf_bias_z.c  Multiplication=Matrix(K*u)  SampleTime=Ts
  Constant : Constant  Value=[0]
  D : Gain  Gain=kalmf_bias_z.d  Multiplication=Matrix(K*u)  SampleTime=Ts
  Demux2 : Demux  Outputs=3
  Mux1 : Mux  Inputs=2
  Mux2 : Mux  Inputs=2
  Sum1 : Sum  Inputs=++|
  Sum2 : Sum  Inputs=++|
  Terminator2 : Terminator
  Unit Delay External IC : simulink/Additional Math & Discrete/Additional Discrete/Unit Delay External IC  SystemSampleTime=-1  tsamp=-1
  z_states_est : Outport  PortDimensions=2
  z_bias : Outport  Port=2  PortDimensions=1
  wires:
  Demux2/2 -> z_states_est/1
  Demux2/1 -> Terminator2/1
  z_states_meas/1 -> Bus Selector1/1, Mux1/2
  thrust_cmd/1 -> Mux1/1
  Mux1/1 -> B/1, D/1
  Unit Delay External IC/1 -> A/1, C/1
  Mux2/1 -> Unit Delay External IC/2
  Constant/1 -> Mux2/2
  A/1 -> Sum1/1
  C/1 -> Sum2/2
  D/1 -> Sum2/1
  B/1 -> Sum1/2
  Sum1/1 -> Unit Delay External IC/1
  Sum2/1 -> Demux2/1
  Bus Selector1/1 -> Mux2/1
  Demux2/3 -> z_bias/1

== system remote/pos controller1/decoupling and rotation/decoupling  ==
  "roll_meas  " : Inport  PortDimensions=1
  "pitch_meas  " : Inport  Port=2  PortDimensions=1
  cmd : Inport  Port=3
  Bus Creator : BusCreator
  Bus Selector3 : BusSelector  OutputSignals=pitch_cmd,roll_cmd,thrust_cmd,yaw_rate_cmd
  Embedded MATLAB Function : Stateflow chart  TreatAsAtomicUnit=on
  g : Constant  Value=g
  mass : Constant  Value=mass
  "cmd_comp  " : Outport
  wires:
  "roll_meas  "/1 -> Embedded MATLAB Function/2(roll_meas)
  "pitch_meas  "/1 -> Embedded MATLAB Function/1(pitch_meas)
  cmd/1 -> Bus Selector3/1
  Bus Selector3/4 -> Bus Creator/4  "<yaw_rate_cmd>"
  Bus Creator/1 -> "cmd_comp  "/1
  Embedded MATLAB Function/3(thrust_comp) -> Bus Creator/3  "thrust_cmd"
  Embedded MATLAB Function/2(roll_cmd_comp) -> Bus Creator/2  "roll_cmd"
  Embedded MATLAB Function/1(pitch_cmd_comp) -> Bus Creator/1  "pitch_cmd"
  Bus Selector3/1 -> Embedded MATLAB Function/3(pitch_cmd)  "<pitch_cmd>"
  Bus Selector3/2 -> Embedded MATLAB Function/4(roll_cmd)  "<roll_cmd>"
  Bus Selector3/3 -> Embedded MATLAB Function/5(thrust)  "<thrust_cmd>"
  mass/1 -> Embedded MATLAB Function/6(m)
  g/1 -> Embedded MATLAB Function/7(g)

== system remote/pos controller1/decoupling and rotation/rotate_to_quat_frame ==
  yaw_meas : Inport
  cmd_comp : Inport  Port=2
  bias : Inport  Port=3
  Bus Creator1 : BusCreator
  Bus Creator2 : BusCreator
  Bus Selector1 : BusSelector  OutputSignals=thrust_bias,yaw_rate_bias
  Bus Selector2 : BusSelector  OutputSignals=pitch_bias,roll_bias
  Bus Selector3 : BusSelector  OutputSignals=pitch_cmd,roll_cmd
  Bus Selector4 : BusSelector  OutputSignals=thrust_cmd,yaw_rate_cmd
  Embedded MATLAB Function : Stateflow chart  TreatAsAtomicUnit=on
  "cmd_rot  " : Outport
  bias_rot : Outport  Port=2
  wires:
  yaw_meas/1 -> Embedded MATLAB Function/1(yaw)
  bias/1 -> Bus Selector2/1, Bus Selector1/1
  Bus Creator1/1 -> bias_rot/1
  Bus Selector2/1 -> Embedded MATLAB Function/4(pitch_bias)  "<pitch_bias>"
  Bus Selector2/2 -> Embedded MATLAB Function/5(roll_bias)  "<roll_bias>"
  Embedded MATLAB Function/3(pitch_bias_rot) -> Bus Creator1/1  "pitch_bias"
  Embedded MATLAB Function/4(roll_bias_rot) -> Bus Creator1/2  "roll_bias"
  Bus Creator2/1 -> "cmd_rot  "/1
  Bus Selector3/2 -> Embedded MATLAB Function/3(roll_cmd)  "<roll_cmd>"
  Bus Selector3/1 -> Embedded MATLAB Function/2(pitch_cmd)  "<pitch_cmd>"
  cmd_comp/1 -> Bus Selector3/1, Bus Selector4/1
  Embedded MATLAB Function/1(pitch_rot) -> Bus Creator2/1  "pitch_cmd"
  Embedded MATLAB Function/2(roll_rot) -> Bus Creator2/2  "roll_cmd"
  Bus Selector4/1 -> Bus Creator2/3  "<thrust_cmd>"
  Bus Selector4/2 -> Bus Creator2/4  "<yaw_rate_cmd>"
  Bus Selector1/1 -> Bus Creator1/3  "<thrust_bias>"
  Bus Selector1/2 -> Bus Creator1/4  "<yaw_rate_bias>"

== matlab function pos controller1/MAIN CONTROL LOOP/x controller MPC FG /runFastGradient ==
  data: TT_PP input double; u_opt output double; LL_PP input double; LL_ref_PP input double; J_star output double; u_buff_out output double; V_init_out output double; MM input double; PP input double; AA_delay input double; BB_delay input double; x input double; X_ref input double; V_max input double; i_min input double; betas input double; L input double; u_buff input double; V_init input double
function [u_opt, J_star, u_buff_out, V_init_out] = fcn(TT_PP, LL_PP,...    
                        LL_ref_PP, MM, PP, AA_delay, BB_delay, x, X_ref,...
                        V_max,i_min, betas, L, u_buff, V_init)

    % ugly, but simulink needs fix output sizes for vectors
    m = 1; % number of outputs u
    delay_steps = 3; % number of delay steps
    N = 30; % prediction horizon
    
    % predict non-delayed state
    if(delay_steps==0)
        x_predicted=x;
    else
        x_predicted=AA_delay*x+BB_delay*u_buff;
    end
    
    
    [J_star, V_star, ~] = ...
        runFastGradient(TT_PP, LL_PP, LL_ref_PP, MM, x_predicted, X_ref, -V_max, V_max, V_init, ...
        i_min, betas, L, []);

    
    % Note: Fast gradient method is implemented in variable V where U = PP * V,
    % so don't forget to backtransform after termination:
    U_star = PP * V_star;

     % save outputs for delayed system
    if(delay_steps==0)
        u_buff_out=0;
    else
        u_buff_out=[u_buff(2:delay_steps,:); U_star(1:m,1)];
    end
 
    % set new initial guess
    V_init_out=[V_star(2:N);0];
    
    u_opt=U_star(1:m,1);

== matlab function pos controller1/decoupling and rotation/decoupling /Embedded MATLAB Function ==
  data: pitch_cmd_comp output double; roll_cmd_comp output double; pitch_meas input double; thrust_comp output double; roll_meas input double; pitch_cmd input double; roll_cmd input double; thrust input double; m input double; g input double
function [pitch_cmd_comp, roll_cmd_comp, thrust_comp]  = fcn(pitch_meas, roll_meas, pitch_cmd, roll_cmd, thrust,m,g)
%#eml

Fx=-m*g*pitch_cmd;
Fy=m*g*roll_cmd;

thrust_comp=thrust/(cos(pitch_meas)*cos(roll_meas));


% pitch_cmd_comp=pitch_cmd;
% roll_cmd_comp=roll_cmd;
% pitch_cmd_comp = atan(Fx/(-thrust_comp));
% roll_cmd_comp = atan(Fy/(thrust_comp));

pitch_cmd_comp = atan(Fx/(-thrust_comp));
roll_cmd_comp = atan(Fy*cos(pitch_meas)/(thrust_comp));

== matlab function create ref1/generate_X_ref ==
  data: x_ref input double; x_dot_ref input double; X_ref output double
function X_ref  = fcn(x_ref, x_dot_ref)
   
pred_horizon=30;

X_ref_temp=[x_ref*ones(1,pred_horizon+1); x_dot_ref*ones(1,pred_horizon+1); zeros(1,pred_horizon+1)];

X_ref=reshape(X_ref_temp,1,[])';

== matlab function pos controller1/MAIN CONTROL LOOP/y controller MPC FG/runFastGradient ==
  data: TT_PP input double; u_opt output double; LL_PP input double; LL_ref_PP input double; J_star output double; u_buff_out output double; V_init_out output double; MM input double; PP input double; AA_delay input double; BB_delay input double; x input double; X_ref input double; V_max input double; i_min input double; betas input double; L input double; u_buff input double; V_init input double
function [u_opt, J_star, u_buff_out, V_init_out] = fcn(TT_PP, LL_PP,...    
                        LL_ref_PP, MM, PP, AA_delay, BB_delay, x, X_ref,...
                        V_max,i_min, betas, L, u_buff, V_init)

    % ugly, but simulink needs fix output sizes for vectors
    m = 1; % number of outputs u
    delay_steps = 3; % number of delay steps
    N = 30; % prediction horizon
    
    % predict non-delayed state
    if(delay_steps==0)
        x_predicted=x;
    else
        x_predicted=AA_delay*x+BB_delay*u_buff;
    end
    
    
    [J_star, V_star, ~] = ...
        runFastGradient(TT_PP, LL_PP, LL_ref_PP, MM, x_predicted, X_ref, -V_max, V_max, V_init, ...
        i_min, betas, L, []);

    
    % Note: Fast gradient method is implemented in variable V where U = PP * V,
    % so don't forget to backtransform after termination:
    U_star = PP * V_star;

     % save outputs for delayed system
    if(delay_steps==0)
        u_buff_out=0;
    else
        u_buff_out=[u_buff(2:delay_steps,:); U_star(1:m,1)];
    end
 
    % set new initial guess
    V_init_out=[V_star(2:N);0];
    
    u_opt=U_star(1:m,1);

== matlab function pos controller1/MAIN CONTROL LOOP/z controller MPC FG/runFastGradient ==
  data: TT_PP input double; u_opt output double; LL_PP input double; LL_ref_PP input double; J_star output double; u_buff_out output double; V_init_out output double; MM input double; PP input double; AA_delay input double; BB_delay input double; x input double; X_ref input double; V_max input double; i_min input double; betas input double; L input double; u_buff input double; V_init input double
function [u_opt, J_star, u_buff_out, V_init_out] = fcn(TT_PP, LL_PP,...    
                        LL_ref_PP, MM, PP, AA_delay, BB_delay, x, X_ref,...
                        V_max,i_min, betas, L, u_buff, V_init)

    % ugly, but simulink needs fix output sizes for vectors
    m = 1; % number of outputs u
    delay_steps = 3; % number of delay steps
    N = 30; % prediction horizon
    
    % predict non-delayed state
    if(delay_steps==0)
        x_predicted=x;
    else
        x_predicted=AA_delay*x+BB_delay*u_buff;
    end
    
    
    [J_star, V_star, ~] = ...
        runFastGradient(TT_PP, LL_PP, LL_ref_PP, MM, x_predicted, X_ref, -V_max, V_max, V_init, ...
        i_min, betas, L, []);

    
    % Note: Fast gradient method is implemented in variable V where U = PP * V,
    % so don't forget to backtransform after termination:
    U_star = PP * V_star;

     % save outputs for delayed system
    if(delay_steps==0)
        u_buff_out=0;
    else
        u_buff_out=[u_buff(2:delay_steps,:); U_star(1:m,1)];
    end
 
    % set new initial guess
    V_init_out=[V_star(2:N);0];
    
    u_opt=U_star(1:m,1);

== matlab function pos controller1/MAIN CONTROL LOOP/yaw controller MPC FG/runFastGradient ==
  data: TT_PP input double; u_opt output double; LL_PP input double; LL_ref_PP input double; J_star output double; u_buff_out output double; V_init_out output double; MM input double; PP input double; AA_delay input double; BB_delay input double; x input double; X_ref input double; V_max input double; i_min input double; betas input double; L input double; u_buff input double; V_init input double
function [u_opt, J_star, u_buff_out, V_init_out] = fcn(TT_PP, LL_PP,...    
                        LL_ref_PP, MM, PP, AA_delay, BB_delay, x, X_ref,...
                        V_max,i_min, betas, L, u_buff, V_init)

    % ugly, but simulink needs fix output sizes for vectors
    m = 1; % number of outputs u
    delay_steps = size(u_buff,1); % number of delay steps
    N = 30; % prediction horizon
    
    % predict non-delayed state
    if(delay_steps==0)
        x_predicted=x;
    else
        x_predicted=AA_delay*x+BB_delay*u_buff;
    end
    
    
    [J_star, V_star, ~] = ...
        runFastGradient(TT_PP, LL_PP, LL_ref_PP, MM, x_predicted, X_ref, -V_max, V_max, V_init, ...
        i_min, betas, L, []);

    
    % Note: Fast gradient method is implemented in variable V where U = PP * V,
    % so don't forget to backtransform after termination:
    U_star = PP * V_star;

     % save outputs for delayed system
    if(delay_steps==0)
        u_buff_out=0;
    else
        u_buff_out=[u_buff(2:delay_steps,:); U_star(1:m,1)];
    end
 
    % set new initial guess
    V_init_out=[V_star(2:N);0];
    
    u_opt=U_star(1:m,1);

== matlab function create ref1/generate_X_ref1 ==
  data: x_ref input double; x_dot_ref input double; X_ref output double
function X_ref  = fcn(x_ref, x_dot_ref)
   
pred_horizon=30;

X_ref_temp=[x_ref*ones(1,pred_horizon+1); x_dot_ref*ones(1,pred_horizon+1); zeros(1,pred_horizon+1)];

X_ref=reshape(X_ref_temp,1,[])';

== matlab function create ref1/generate_X_ref2 ==
  data: x_ref input double; x_dot_ref input double; X_ref output double
function X_ref  = fcn(x_ref, x_dot_ref)
   
pred_horizon=30;

X_ref_temp=[x_ref*ones(1,pred_horizon+1); x_dot_ref*ones(1,pred_horizon+1)];

X_ref=reshape(X_ref_temp,1,[])';

== matlab function create ref1/generate_X_ref3 ==
  data: x_ref input double; x_dot_ref input double; X_ref output double
function X_ref  = fcn(x_ref, x_dot_ref)
   
pred_horizon=30;

X_ref_temp=[x_ref*ones(1,pred_horizon+1); x_dot_ref*ones(1,pred_horizon+1)];

X_ref=reshape(X_ref_temp,1,[])';
